simulink model "examplePumpConst"  (Simulink 8.2)
settings: Solver=ode45  StartTime=0.0  StopTime=240  RelTol=1e-3
libraries: carnot x2
settings Model: Creator=drhf  LastModifiedBy=drhf
settings DataIOCC: SignalLoggingSaveFormat=Dataset
settings DebuggingCC: FcnCallInpInsideContextMsg=EnableAllAsError

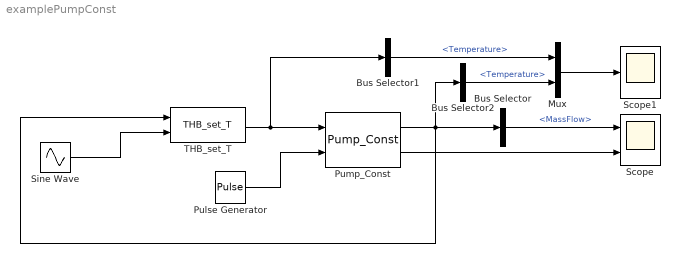
== system examplePumpConst ==
  Bus Selector : BusSelector  OutputSignals=MassFlow
  Bus Selector1 : BusSelector  OutputSignals=Temperature
  Bus Selector2 : BusSelector  OutputSignals=Temperature
  Mux : Mux  Inputs=2
  Pulse Generator : DiscretePulseGenerator  PulseType=Time based  Period=120  PulseWidth=50
  Pump_Const : carnot/Hydraulics/Pump_Const  mdotmax=1200/3600  dia=0.0157  power=30  p0=3e5  fluid_id=Water  mix=0  UA=3  mcp=4000  tamb=20
  Scope : Scope  NumInputPorts=2
      settings: YMin=-5~-5  YMax=5~5
  Scope1 : Scope
  Sine Wave : Sin  Amplitude=5  Bias=20  Frequency=2*pi/240  SampleTime=0
  THB_set_T : carnot/Source/Simple/THB_set_T
  wires:
  Pump_Const/1 -> THB_set_T/1, Bus Selector/1, Bus Selector2/1
  THB_set_T/1 -> Pump_Const/1, Bus Selector1/1
  Pulse Generator/1 -> Pump_Const/2
  Pump_Const/2 -> Scope/2
  Bus Selector/1 -> Scope/1  "<MassFlow>"
  Bus Selector1/1 -> Mux/1  "<Temperature>"
  Bus Selector2/1 -> Mux/2  "<Temperature>"
  Mux/1 -> Scope1/1
  Sine Wave/1 -> THB_set_T/2
